simulink model "Lab_1"  (R2020a)
settings: Solver=FixedStepAuto  StartTime=0.0  StopTime=10.0  FixedStep=1e-3  RelTol=1e-3  EnableMultiTasking=on
libraries: frdmk64flib x1
settings Model: ExtModeTrigDuration=5  Creator=Ethan  LastModifiedBy=Ethan
settings OptimizationCC: EnhancedBackFolding=on  PassReuseOutputArgsAs=Individual arguments  ZeroExternalMemoryAtStartup=off  ZeroInternalMemoryAtStartup=off  MaxStackSize=64  OptimizeBlockOrder=speed  DifferentSizesBufferReuse=on  OptimizationCustomize=off  EfficientTunableParamExpr=on
settings DebuggingCC: ParameterTunabilityLossMsg=error
settings HardwareCC: ProdBitPerPointer=32  ProdBitPerSizeT=32  ProdBitPerPtrDiffT=32  ProdLargestAtomicInteger=Long  ProdLargestAtomicFloat=Double  ProdWordSize=32  ProdHWDeviceType=ARM Compatible->ARM Cortex
settings SFSimCC: MATLABDynamicMemAlloc=off
settings RTWCC: SystemTargetFile=ert.tlc  HardwareBoard=NXP FRDM-K64F  TemplateMakefile=ert_default_tmf  Toolchain=GNU Tools for ARM Embedded Processors
settings CodeAppCC: ForceParamTrailComments=on  IgnoreCustomStorageClasses=off  OperatorAnnotations=on  SimulinkDataObjDesc=on  SFDataObjDesc=on  InsertBlockDesc=on

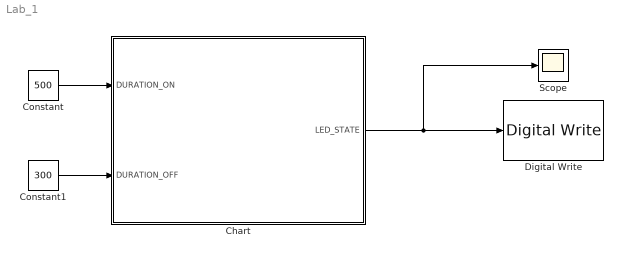
== system Lab_1 ==
  Chart : Stateflow chart  TreatAsAtomicUnit=on
  Constant : Constant  Value=500  OutDataTypeStr=int16
  Constant1 : Constant  Value=300  OutDataTypeStr=int16
  Digital Write : frdmk64flib/Digital Write  Whichpin=RED_LED
  Scope : Scope
  wires:
  Chart/1(LED_STATE) -> Scope/1, Digital Write/1
  Constant/1 -> Chart/1(DURATION_ON)
  Constant1/1 -> Chart/2(DURATION_OFF)

== stateflow chart Lab_1/Chart ==
  state LED_ON
    entry:
    LED_STATE= true;
  state LED_OFF
    entry:
    LED_STATE= false;
  (default) -> LED_ON
  LED_ON -> LED_OFF : after(DURATION_ON, msec)
  LED_OFF -> LED_ON : after(DURATION_OFF, msec)
  data: DURATION_ON input int16; DURATION_OFF input int16; LED_STATE output boolean
